simulink model "corner_light_model"  (R2020a)
settings: Solver=FixedStepDiscrete  StartTime=0.0  StopTime=10.0  RelTol=1e-3
model workspace (MAT data in the model file):
  Als_Mode = Simulink.Signal
  Als_Mode.DataType = 'Enum: Corner_light'
  Als_Mode.Dimensions = -1
  Als_Mode.DimensionsMode = 'auto'
  Als_Mode.Complexity = 'auto'
  Als_Mode.SampleTime = -1
  Als_Mode.SamplingMode = 'auto'
  Als_Mode_off = Simulink.Parameter
  Als_Mode_off.DataType = 'Enum: Corner_light'
  Als_Mode_off.Dimensions = [0 0]
  Als_Mode_on = Simulink.Parameter
  Als_Mode_on.DataType = 'Enum: Corner_light'
  Als_Mode_on.Dimensions = [0 0]
  Corner_Light_Off = Simulink.Parameter
  Corner_Light_Off.DataType = 'Enum: Corner_light'
  Corner_Light_Off.Dimensions = [0 0]
  Corner_Light_On = Simulink.Parameter
  Corner_Light_On.DataType = 'Enum: Corner_light'
  Corner_Light_On.Dimensions = [0 0]
  Ignition = Simulink.Signal
  Ignition.DataType = 'Enum: Corner_light'
  Ignition.Dimensions = -1
  Ignition.DimensionsMode = 'auto'
  Ignition.Complexity = 'auto'
  Ignition.SampleTime = -1
  Ignition.SamplingMode = 'auto'
  Ignition_off = Simulink.Parameter
  Ignition_off.DataType = 'Enum: Corner_light'
  Ignition_off.Dimensions = [0 0]
  Ignition_on = Simulink.Parameter
  Ignition_on.DataType = 'Enum:Corner_light'
  Ignition_on.Dimensions = [0 0]
  Left_Corner_Light_On = Simulink.Parameter
  Left_Corner_Light_On.DataType = 'Enum: Corner_light'
  Left_Corner_Light_On.Dimensions = [0 0]
  Left_InnerWheel_Angle = Simulink.Parameter
  Left_InnerWheel_Angle.Value = 0
  Left_InnerWheel_Angle.DataType = 'uint16'
  Left_InnerWheel_Angle.Dimensions = [1 1]
  Right_Corner_Light_On = Simulink.Parameter
  Right_Corner_Light_On.DataType = 'Enum: Corner_light'
  Right_Corner_Light_On.Dimensions = [0 0]
  Right_InnerWheel_Angle = Simulink.Parameter
  Right_InnerWheel_Angle.Value = 0
  Right_InnerWheel_Angle.DataType = 'uint8'
  Right_InnerWheel_Angle.Dimensions = [1 1]
  Speed = Simulink.Signal
  Speed.DataType = 'uint8'
  Speed.Dimensions = -1
  Speed.DimensionsMode = 'auto'
  Speed.Complexity = 'auto'
  Speed.SampleTime = -1
  Speed.SamplingMode = 'auto'
  Visual = Simulink.Signal
  Visual.DataType = 'Enum: Corner_light'
  Visual.Dimensions = -1
  Visual.DimensionsMode = 'auto'
  Visual.Complexity = 'auto'
  Visual.SampleTime = -1
  Visual.SamplingMode = 'auto'
  Visual_Day_time = Simulink.Parameter
  Visual_Day_time.DataType = 'Enum: Corner_light'
  Visual_Day_time.Dimensions = [0 0]
  Visual_Night_time = Simulink.Parameter
  Visual_Night_time.DataType = 'Enum: Corner_light'
  Visual_Night_time.Dimensions = [0 0]
  speed = Simulink.Parameter
  speed.Value = 40
  speed.DataType = 'uint16'
  speed.Dimensions = [1 1]
undefined symbols (not defined in the file or in its folder): Corner_light
libraries: simulink x10
settings Model: DataDictionary=Corner_Light_dd.sldd  OrderedModelArguments=off  Creator=hp  LastModifiedBy=hp
settings OptimizationCC: DefaultParameterBehavior=Inlined  EnhancedBackFolding=on  PassReuseOutputArgsAs=Individual arguments  ZeroExternalMemoryAtStartup=off  ZeroInternalMemoryAtStartup=off  OptimizeBlockOrder=speed  DifferentSizesBufferReuse=on  OptimizationCustomize=off  EfficientTunableParamExpr=on
settings DebuggingCC: ParameterTunabilityLossMsg=error
settings SFSimCC: MATLABDynamicMemAlloc=off
settings RTWCC: SystemTargetFile=ert.tlc  TemplateMakefile=ert_default_tmf  Toolchain=MinGW64 | gmake (64-bit Windows)
settings CodeAppCC: ForceParamTrailComments=on  IgnoreCustomStorageClasses=off  OperatorAnnotations=on  SimulinkDataObjDesc=on  SFDataObjDesc=on  InsertBlockDesc=on
settings ERTTargetCC: TargetLangStandard=C99 (ISO)  GenerateSampleERTMain=on  InlinedParameterPlacement=NonHierarchical  ERTCustomFileTemplate=example_file_process.tlc

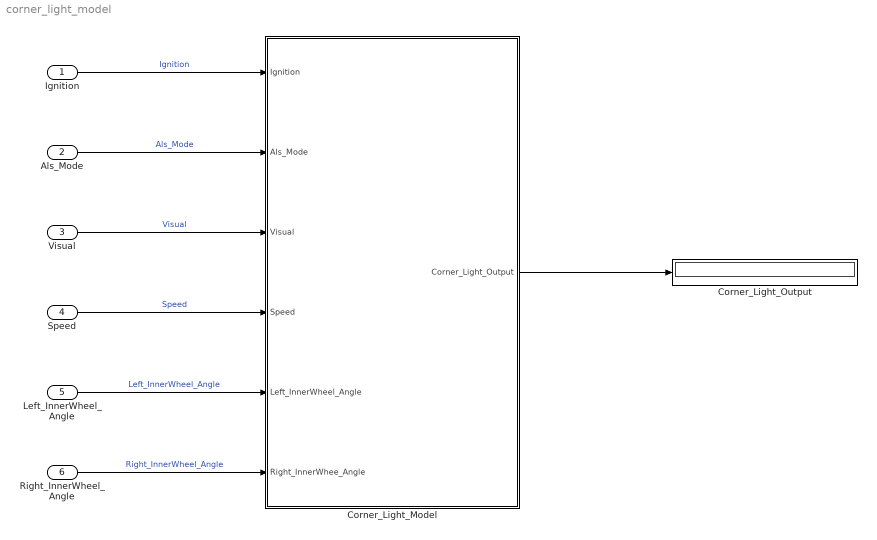
== system corner_light_model ==
  Ignition : Inport
  Als_Mode : Inport  Port=2
  Visual : Inport  Port=3
  Speed : Inport  Port=4
  Left_InnerWheel_Angle : Inport  Port=5
  Right_InnerWheel_Angle : Inport  Port=6
  Corner_Light_Model : Subsystem
  Corner_Light_Output : Display
  wires:
  Ignition/1 -> Corner_Light_Model/1(Ignition)  "Ignition"
  Corner_Light_Model/1(Corner_Light_Output) -> Corner_Light_Output/1
  Speed/1 -> Corner_Light_Model/4(Speed)  "Speed"
  Als_Mode/1 -> Corner_Light_Model/2(Als_Mode)  "Als_Mode"
  Visual/1 -> Corner_Light_Model/3(Visual)  "Visual"
  Left_InnerWheel_Angle/1 -> Corner_Light_Model/5(Left_InnerWheel_Angle)  "Left_InnerWheel_Angle"
  Right_InnerWheel_Angle/1 -> Corner_Light_Model/6(Right_InnerWhee_Angle)  "Right_InnerWheel_Angle"

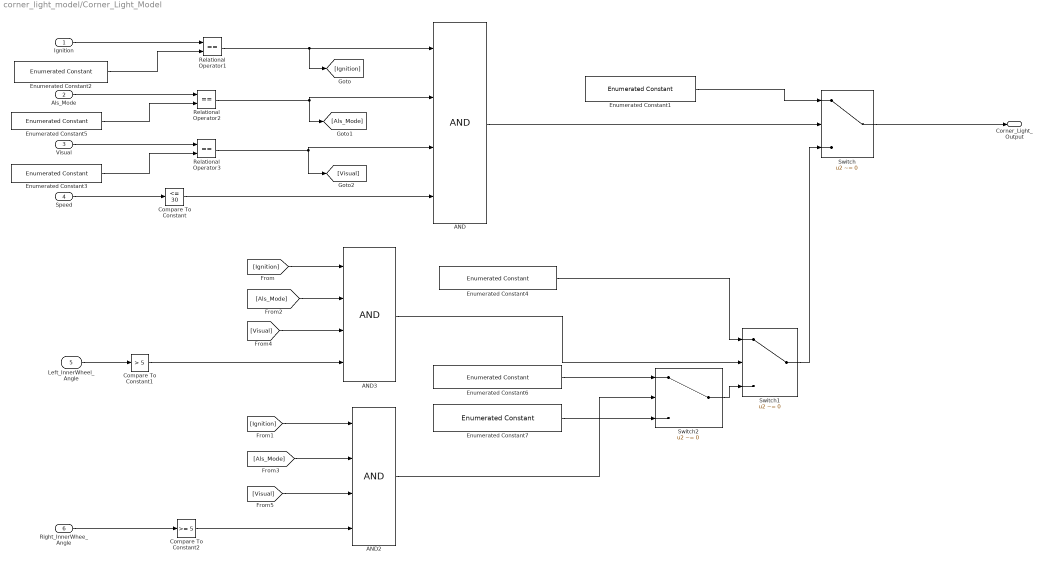
== system corner_light_model/Corner_Light_Model ==
  Ignition : Inport
  Als_Mode : Inport  Port=2
  Visual : Inport  Port=3
  Speed : Inport  Port=4
  Left_InnerWheel_Angle : Inport  Port=5
  Right_InnerWhee_Angle : Inport  Port=6
  AND : Logic  Inputs=4  AllPortsSameDT=off  OutDataTypeStr=boolean
  AND2 : Logic  Inputs=4  AllPortsSameDT=off  OutDataTypeStr=boolean
  AND3 : Logic  Inputs=4  AllPortsSameDT=off  OutDataTypeStr=boolean
  Compare To Constant : simulink/Logic and Bit Operations/Compare To Constant  relop=<=  const=30  OutDataTypeStr=boolean
  Compare To Constant1 : simulink/Logic and Bit Operations/Compare To Constant  relop=>  const=5  OutDataTypeStr=uint8
  Compare To Constant2 : simulink/Logic and Bit Operations/Compare To Constant  relop=>=  const=5  OutDataTypeStr=boolean
  Enumerated Constant1 : simulink/Sources/Enumerated Constant  OutDataTypeStr=Enum:Corner_light  Value=Corner_light.Corner_Light_On  SampleTime=inf
  Enumerated Constant2 : simulink/Sources/Enumerated Constant  OutDataTypeStr=Enum:Corner_light  Value=Corner_light.Ignition_on  SampleTime=inf
  Enumerated Constant3 : simulink/Sources/Enumerated Constant  OutDataTypeStr=Enum:Corner_light  Value=Corner_light.Visual_Night_time  SampleTime=inf
  Enumerated Constant4 : simulink/Sources/Enumerated Constant  OutDataTypeStr=Enum:Corner_light  Value=Corner_light.Left_Corner_Light_On  SampleTime=inf
  Enumerated Constant5 : simulink/Sources/Enumerated Constant  OutDataTypeStr=Enum:Corner_light  Value=Corner_light.Als_Mode_on  SampleTime=inf
  Enumerated Constant6 : simulink/Sources/Enumerated Constant  OutDataTypeStr=Enum:Corner_light  Value=Corner_light.Right_Corner_Light_On  SampleTime=inf
  Enumerated Constant7 : simulink/Sources/Enumerated Constant  OutDataTypeStr=Enum:Corner_light  Value=Corner_light.Corner_Lights_Off  SampleTime=inf
  Relational Operator1 : RelationalOperator  Operator===  OutDataTypeStr=boolean  RndMeth=Simplest
  Relational Operator2 : RelationalOperator  Operator===  OutDataTypeStr=boolean  RndMeth=Simplest
  Relational Operator3 : RelationalOperator  Operator===  OutDataTypeStr=boolean  RndMeth=Simplest
  Switch : Switch  Criteria=u2 ~= 0
  Switch1 : Switch  Criteria=u2 ~= 0
  Switch2 : Switch  Criteria=u2 ~= 0
  Corner_Light_Output : Outport
  wires:
  Speed/1 -> Compare To Constant/1
  Ignition/1 -> Relational Operator1/1
  Enumerated Constant2/1 -> Relational Operator1/2
  Visual/1 -> Relational Operator3/1
  Als_Mode/1 -> Relational Operator2/1
  Relational Operator1/1 -> [Ignition], AND/1
  Enumerated Constant1/1 -> Switch/1
  Switch2/1 -> Switch1/3
  Enumerated Constant4/1 -> Switch1/1
  Relational Operator2/1 -> [Als_Mode], AND/2
  Relational Operator3/1 -> [Visual], AND/3
  Switch1/1 -> Switch/3
  AND2/1 -> Switch2/2
  Switch/1 -> Corner_Light_Output/1
  AND3/1 -> Switch1/2
  AND/1 -> Switch/2
  [Ignition] -> AND3/1
  [Ignition] -> AND2/1
  [Als_Mode] -> AND2/2
  [Visual] -> AND2/3
  [Als_Mode] -> AND3/2
  [Visual] -> AND3/3
  Right_InnerWhee_Angle/1 -> Compare To Constant2/1
  Left_InnerWheel_Angle/1 -> Compare To Constant1/1
  Compare To Constant/1 -> AND/4
  Compare To Constant2/1 -> AND2/4
  Compare To Constant1/1 -> AND3/4
  Enumerated Constant5/1 -> Relational Operator2/2
  Enumerated Constant3/1 -> Relational Operator3/2
  Enumerated Constant6/1 -> Switch2/1
  Enumerated Constant7/1 -> Switch2/3
